simulink model "example_of_sign_block_and_PWM_block"  (R2021a)
settings: Solver=VariableStepAuto  StartTime=0.0  StopTime=10.0  RelTol=1e-3
libraries: simulink x1
settings Model: Creator=YasserNet  LastModifiedBy=YasserNet

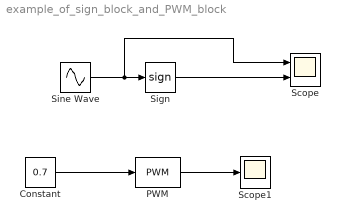
== system example_of_sign_block_and_PWM_block ==
  Constant : Constant  Value=0.7
  PWM : simulink/Discontinuities/PWM  DisableCoverage=on  Period=1  DisallowZeroDutyCycle=off  RunAtFixedTimeIntervals=off  SampleTime=0.1
  Scope : Scope  NumInputPorts=2
  Scope1 : Scope
  Sign : Signum
  Sine Wave : Sin  Frequency=2*pi  SampleTime=0
  wires:
  Sign/1 -> Scope/2
  Sine Wave/1 -> Scope/1, Sign/1
  Constant/1 -> PWM/1
  PWM/1 -> Scope1/1
